simulink model "ControlCore"  (R2022a)
settings: Solver=VariableStepAuto  StartTime=0.0  StopTime=10.0  RelTol=1e-3
InitFcn:
  | master_init;
libraries: CarMaker4SL x12
settings Model: Creator=krisz  LastModifiedBy=krisz

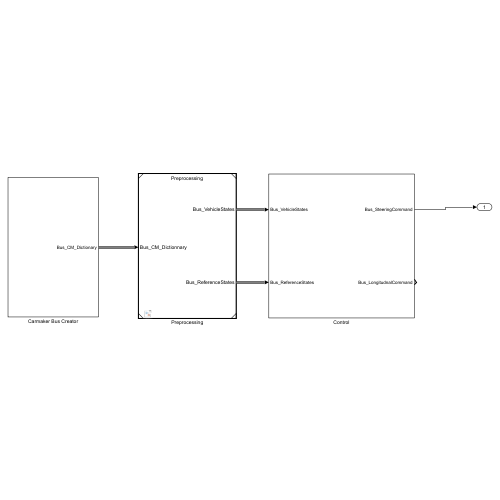
[thumbnail: Simulink's stored preview of the top-level diagram]
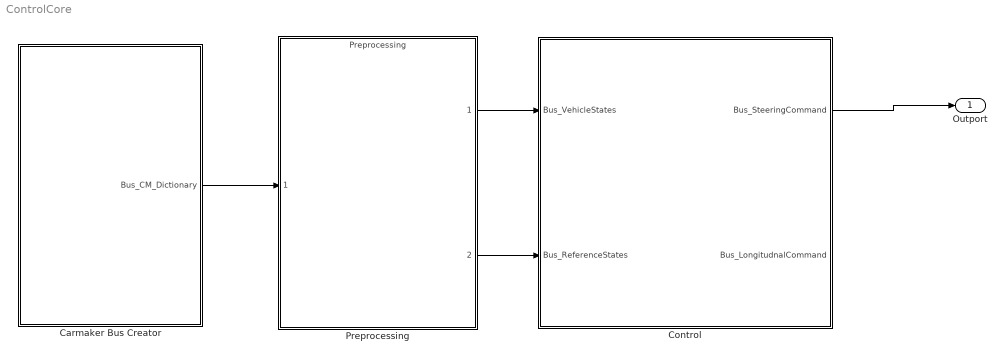
== system ControlCore ==
  Carmaker Bus Creator : Subsystem
  Control : Subsystem
  Preprocessing : ModelReference  ModelNameDialog=Preprocessing.slx  SimulationMode=Normal  ModelReferenceVersion=1.6
  Outport : Outport
  wires:
  Carmaker Bus Creator/1(Bus_CM_Dictionary) -> Preprocessing/1
  Preprocessing/1 -> Control/1(Bus_VehicleStates)
  Preprocessing/2 -> Control/2(Bus_ReferenceStates)
  Control/1(Bus_SteeringCommand) -> Outport/1

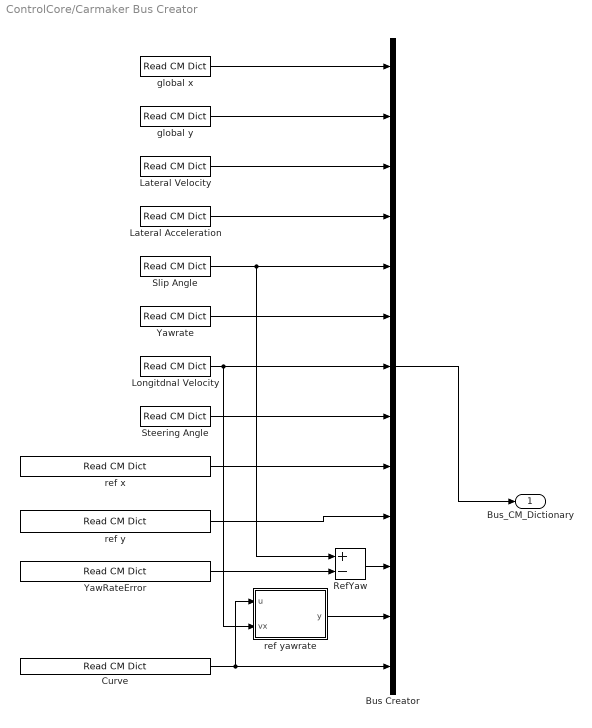
== system ControlCore/Carmaker Bus Creator ==
  Bus Creator : BusCreator  Inputs=13  OutDataTypeStr=Bus: Bus_CM_Dictionary
      settings: InheritFromInputs=off
  Curve : CarMaker4SL/Read CM Dict  xname=Sensor.Road.VehSensor_0.Path.CurveXY  xsync=off  xstime=Continuous
  Lateral Acceleration : CarMaker4SL/Read CM Dict  xname=Car.ay  xsync=off  xstime=Continuous
  Lateral Velocity : CarMaker4SL/Read CM Dict  xname=Car.vy  xsync=off  xstime=Continuous
  Longitdnal Velocity : CarMaker4SL/Read CM Dict  xname=Car.vx  xsync=off  xstime=Continuous
  RefYaw : Sum  Inputs=+-
  Slip Angle : CarMaker4SL/Read CM Dict  xname=Car.Yaw  xsync=off  xstime=Continuous
  Steering Angle : CarMaker4SL/Read CM Dict  xname=Vhcl.Steer.Ang  xsync=off  xstime=Continuous
  YawRateError : CarMaker4SL/Read CM Dict  xname=Sensor.Road.VehSensor_0.Path.DevAng  xsync=off  xstime=Continuous
  Yawrate : CarMaker4SL/Read CM Dict  xname=Car.YawRate  xsync=off  xstime=Continuous
  global x : CarMaker4SL/Read CM Dict  xname=Car.tx  xsync=off  xstime=Continuous
  global y : CarMaker4SL/Read CM Dict  xname=Car.ty  xsync=off  xstime=Continuous
  ref x : CarMaker4SL/Read CM Dict  xname=Sensor.Road.VehSensor_0.Path.tx  xsync=off  xstime=Continuous
  ref y : CarMaker4SL/Read CM Dict  xname=Sensor.Road.VehSensor_0.Path.ty  xsync=off  xstime=Continuous
  ref yawrate : MATLAB Function  TreatAsAtomicUnit=on
  Bus_CM_Dictionary : Outport  OutDataTypeStr=Bus: Bus_CM_Dictionary
  wires:
  Bus Creator/1 -> Bus_CM_Dictionary/1
  Slip Angle/1 -> RefYaw/1, Bus Creator/5
  Longitdnal Velocity/1 -> ref yawrate/2(vx), Bus Creator/7
  Curve/1 -> Bus Creator/13, ref yawrate/1(u)
  YawRateError/1 -> RefYaw/2
  global x/1 -> Bus Creator/1
  global y/1 -> Bus Creator/2
  Lateral Velocity/1 -> Bus Creator/3
  Lateral Acceleration/1 -> Bus Creator/4
  Yawrate/1 -> Bus Creator/6
  Steering Angle/1 -> Bus Creator/8
  ref yawrate/1(y) -> Bus Creator/12
  RefYaw/1 -> Bus Creator/11
  ref x/1 -> Bus Creator/9
  ref y/1 -> Bus Creator/10

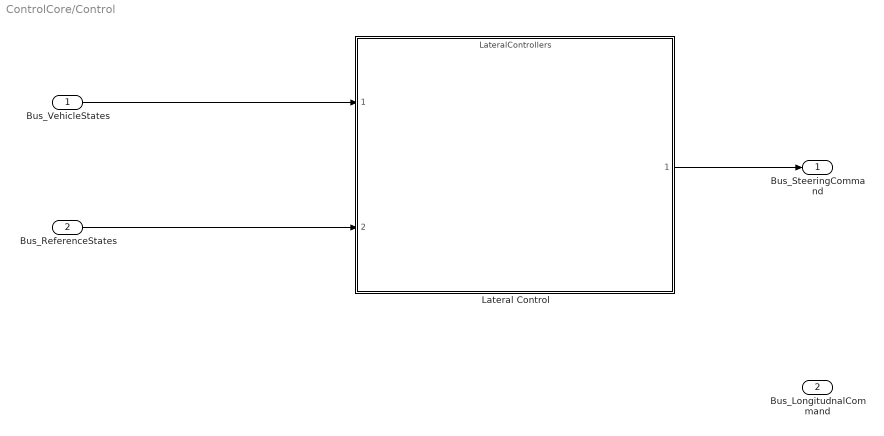
== system ControlCore/Control ==
  Bus_VehicleStates : Inport  OutDataTypeStr=Bus: bus_VehicleStates
  Bus_ReferenceStates : Inport  Port=2  OutDataTypeStr=Bus: bus_ReferenceStates
  Lateral Control : ModelReference  ModelNameDialog=LateralControllers.slx  SimulationMode=Normal  ModelReferenceVersion=1.7
  Bus_SteeringCommand : Outport
  Bus_LongitudnalCommand : Outport  Port=2
  wires:
  Lateral Control/1 -> Bus_SteeringCommand/1
  Bus_VehicleStates/1 -> Lateral Control/1
  Bus_ReferenceStates/1 -> Lateral Control/2

== matlab function ControlCore/Carmaker Bus Creator/ref yawrate ==
  data: u input; y output; vx input
function y = fcn(u,vx)

y = u*vx;
